simulink model "CL_Master"  (R2020b)
settings: configuration reference "VLS_Standard_Configuration" (kept outside this file)
model workspace (MAT data in the model file):
  M_combineLogic = Simulink.Parameter
  M_combineLogic.Value = [0; 1; 0; 1]
  M_combineLogic.DataType = 'boolean'
  M_combineLogic.Dimensions = [4 1]
undefined symbols (not defined in the file): C_CL_Ti_Speed_Hystresis, C_CL_Ti_Speed_Threshold, C_ClLeftSideTable_Alpha1, C_ClLeftSideTable_Alpha2, C_ClRightSideTable_Alpha1, C_ClRightSideTable_Alpha2, C_ClSpeedCurve, C_ClTableSize, C_Cuvre_StWhAngPriority, C_TiActiveCycle
libraries: Cl_Lib x1
settings Model: DataDictionary=CL_MasterDD.sldd  EnableAccessToBaseWorkspace=off  Creator=mteama  LastModifiedBy=mtarek-a
settings ConfigSetRef: SourceName=VLS_Standard_Configuration

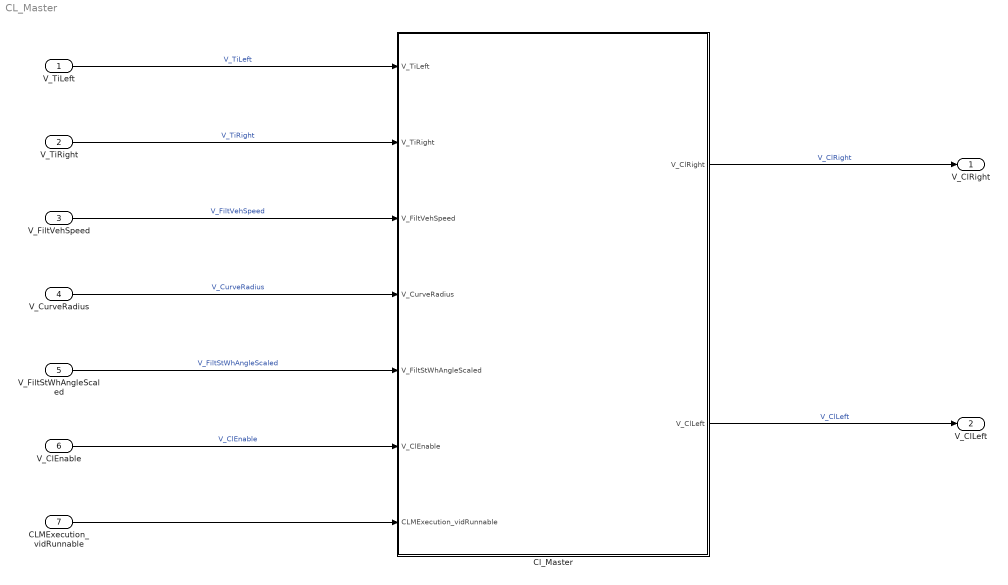
== system CL_Master ==
  V_TiLeft : Inport
  V_TiRight : Inport  Port=2
  V_FiltVehSpeed : Inport  Port=3
  V_CurveRadius : Inport  Port=4
  V_FiltStWhAngleScaled : Inport  Port=5
  V_ClEnable : Inport  Port=6
  CLMExecution_vidRunnable : Inport  Port=7  SampleTime=0.02  OutputFunctionCall=on
  Cl_Master : Subsystem
  V_ClRight : Outport
  V_ClLeft : Outport  Port=2
  wires:
  V_TiLeft/1 -> Cl_Master/1(V_TiLeft)  "V_TiLeft"
  V_TiRight/1 -> Cl_Master/2(V_TiRight)  "V_TiRight"
  V_FiltVehSpeed/1 -> Cl_Master/3(V_FiltVehSpeed)  "V_FiltVehSpeed"
  V_CurveRadius/1 -> Cl_Master/4(V_CurveRadius)  "V_CurveRadius"
  CLMExecution_vidRunnable/1 -> Cl_Master/7(CLMExecution_vidRunnable)
  V_FiltStWhAngleScaled/1 -> Cl_Master/5(V_FiltStWhAngleScaled)  "V_FiltStWhAngleScaled"
  Cl_Master/2(V_ClLeft) -> V_ClLeft/1  "V_ClLeft"
  Cl_Master/1(V_ClRight) -> V_ClRight/1  "V_ClRight"
  V_ClEnable/1 -> Cl_Master/6(V_ClEnable)  "V_ClEnable"

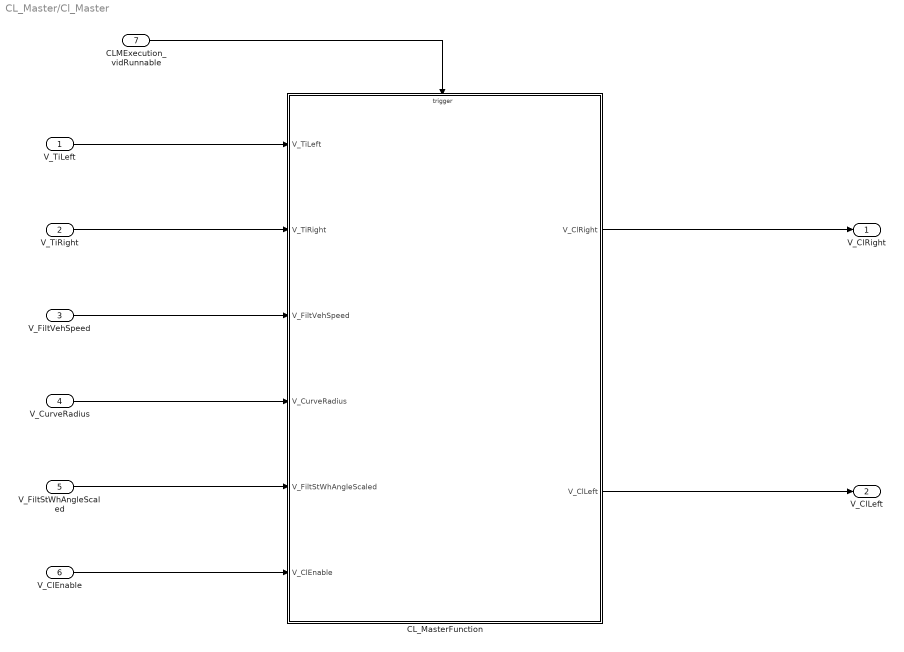
== system CL_Master/Cl_Master ==
  V_TiLeft : Inport
  V_TiRight : Inport  Port=2
  V_FiltVehSpeed : Inport  Port=3
  V_CurveRadius : Inport  Port=4
  V_FiltStWhAngleScaled : Inport  Port=5
  V_ClEnable : Inport  Port=6
  CLMExecution_vidRunnable : Inport  Port=7  SampleTime=0.02  OutputFunctionCall=on
  CL_MasterFunction : Subsystem
  V_ClRight : Outport
  V_ClLeft : Outport  Port=2
  wires:
  V_FiltVehSpeed/1 -> CL_MasterFunction/3(V_FiltVehSpeed)
  V_TiLeft/1 -> CL_MasterFunction/1(V_TiLeft)
  V_TiRight/1 -> CL_MasterFunction/2(V_TiRight)
  CLMExecution_vidRunnable/1 -> CL_MasterFunction/Trigger
  V_CurveRadius/1 -> CL_MasterFunction/4(V_CurveRadius)
  V_FiltStWhAngleScaled/1 -> CL_MasterFunction/5(V_FiltStWhAngleScaled)
  CL_MasterFunction/1(V_ClRight) -> V_ClRight/1
  CL_MasterFunction/2(V_ClLeft) -> V_ClLeft/1
  V_ClEnable/1 -> CL_MasterFunction/6(V_ClEnable)

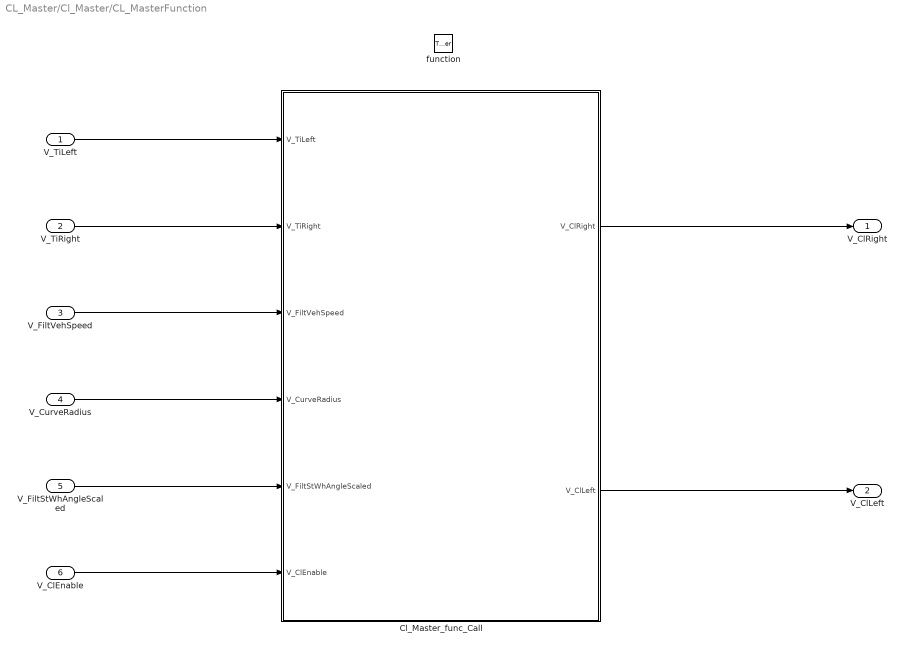
== system CL_Master/Cl_Master/CL_MasterFunction ==
  V_TiLeft : Inport
  V_TiRight : Inport  Port=2
  V_FiltVehSpeed : Inport  Port=3
  V_CurveRadius : Inport  Port=4
  V_FiltStWhAngleScaled : Inport  Port=5
  V_ClEnable : Inport  Port=6
  function : TriggerPort  TriggerType=function-call  VariantControl=Variant
  Cl_Master_func_Call : Subsystem
  V_ClRight : Outport
  V_ClLeft : Outport  Port=2
  wires:
  V_FiltVehSpeed/1 -> Cl_Master_func_Call/3(V_FiltVehSpeed)
  V_CurveRadius/1 -> Cl_Master_func_Call/4(V_CurveRadius)
  V_TiLeft/1 -> Cl_Master_func_Call/1(V_TiLeft)
  V_TiRight/1 -> Cl_Master_func_Call/2(V_TiRight)
  V_FiltStWhAngleScaled/1 -> Cl_Master_func_Call/5(V_FiltStWhAngleScaled)
  Cl_Master_func_Call/2(V_ClLeft) -> V_ClLeft/1
  Cl_Master_func_Call/1(V_ClRight) -> V_ClRight/1
  V_ClEnable/1 -> Cl_Master_func_Call/6(V_ClEnable)

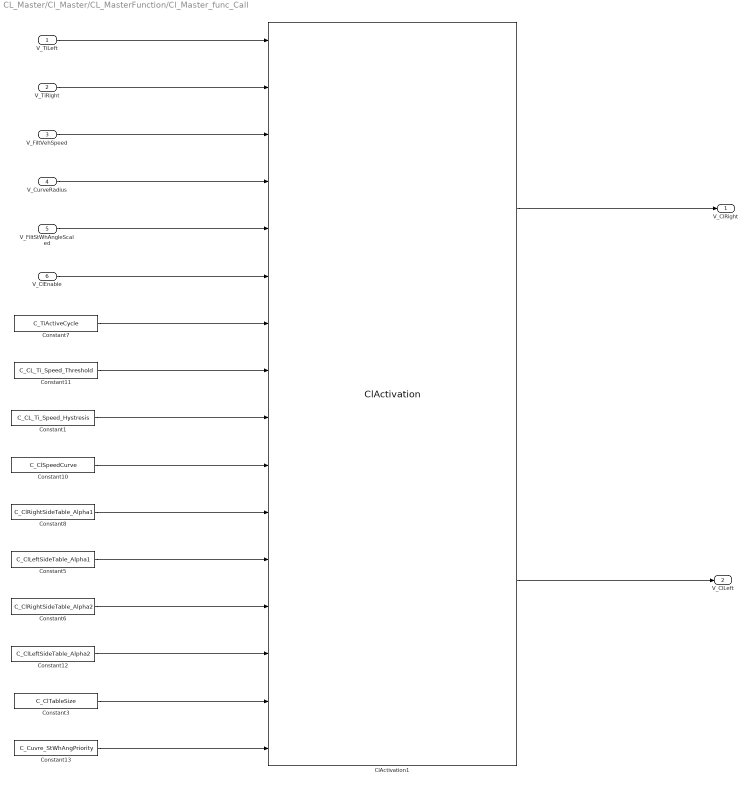
== system CL_Master/Cl_Master/CL_MasterFunction/Cl_Master_func_Call ==
  V_TiLeft : Inport
  V_TiRight : Inport  Port=2
  V_FiltVehSpeed : Inport  Port=3
  V_CurveRadius : Inport  Port=4
  V_FiltStWhAngleScaled : Inport  Port=5
  V_ClEnable : Inport  Port=6
  ClActivation1 : Cl_Lib/ClActivation  SystemSampleTime=-1  VariantActivationTime=update diagram  Latency=0  AutoFrameSizeCalculation=off
  Constant1 : Constant  Value=C_CL_Ti_Speed_Hystresis
  Constant10 : Constant  Value=C_ClSpeedCurve
  Constant11 : Constant  Value=C_CL_Ti_Speed_Threshold
  Constant12 : Constant  Value=C_ClLeftSideTable_Alpha2
  Constant13 : Constant  Value=C_Cuvre_StWhAngPriority
  Constant3 : Constant  Value=C_ClTableSize
  Constant5 : Constant  Value=C_ClLeftSideTable_Alpha1
  Constant6 : Constant  Value=C_ClRightSideTable_Alpha2
  Constant7 : Constant  Value=C_TiActiveCycle
  Constant8 : Constant  Value=C_ClRightSideTable_Alpha1
  V_ClRight : Outport
  V_ClLeft : Outport  Port=2
  wires:
  V_TiRight/1 -> ClActivation1/2
  V_FiltVehSpeed/1 -> ClActivation1/3
  ClActivation1/1 -> V_ClRight/1
  V_CurveRadius/1 -> ClActivation1/4
  V_TiLeft/1 -> ClActivation1/1
  V_FiltStWhAngleScaled/1 -> ClActivation1/5
  ClActivation1/2 -> V_ClLeft/1
  Constant13/1 -> ClActivation1/16
  Constant3/1 -> ClActivation1/15
  Constant12/1 -> ClActivation1/14
  V_ClEnable/1 -> ClActivation1/6
  Constant5/1 -> ClActivation1/12
  Constant8/1 -> ClActivation1/11
  Constant6/1 -> ClActivation1/13
  Constant10/1 -> ClActivation1/10
  Constant1/1 -> ClActivation1/9
  Constant11/1 -> ClActivation1/8
  Constant7/1 -> ClActivation1/7
